simulink model "Q2_Vehicle_Steering_System"  (R2020a)
settings: Solver=VariableStepAuto  StartTime=0.0  StopTime=100  MaxStep=0.01  RelTol=1e-3
values from neighbouring files (symbols this model uses):
  A = [[0,1];[0,0]]    [Variables.m]
  B = [0.4; 1]    [Variables.m]
  C = eye(2)    [Variables.m]
  D = [0;0]    [Variables.m]
  K = [0.2500, 1.3]    [Variables.m]
  Kr = 0.25    [Variables.m]
  L = [2,1]    [Variables.m]
settings Model: Creator=Ajita Shree  LastModifiedBy=Ajita Shree

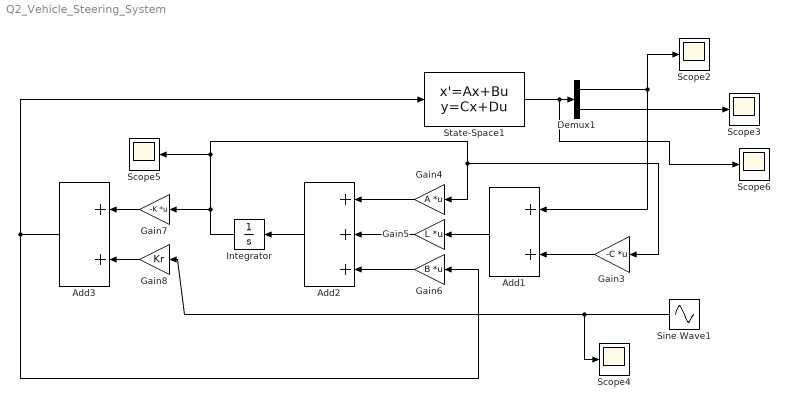
== system Q2_Vehicle_Steering_System ==
  Add1 : Sum
  Add2 : Sum  Inputs=+++
  Add3 : Sum
  Demux1 : Demux  Outputs=2
  Gain3 : Gain  Gain=-C  Multiplication=Matrix(K*u)
  Gain4 : Gain  Gain=A  Multiplication=Matrix(K*u)
  Gain5 : Gain  Gain=L  Multiplication=Matrix(K*u)
  Gain6 : Gain  Gain=B  Multiplication=Matrix(K*u)
  Gain7 : Gain  Gain=-K  Multiplication=Matrix(K*u)
  Gain8 : Gain  Gain=Kr
  Integrator : Integrator
  Scope{2..6} (5 alike) : Scope
  Sine Wave1 : Sin  Frequency=0.5  SampleTime=0
  State-Space1 : StateSpace  A=A  B=B  C=C  D=D  InitialCondition=0
  wires:
  State-Space1/1 -> Scope6/1, Demux1/1
  Demux1/1 -> Add1/1, Scope2/1
  Demux1/2 -> Scope3/1
  Gain4/1 -> Add2/1
  Gain5/1 -> Add2/2
  Gain6/1 -> Add2/3
  Add2/1 -> Integrator/1
  Integrator/1 -> Gain7/1, Gain4/1, Gain3/1, Scope5/1
  Gain3/1 -> Add1/2
  Add1/1 -> Gain5/1
  Add3/1 -> State-Space1/1, Gain6/1
  Gain7/1 -> Add3/1
  Gain8/1 -> Add3/2
  Sine Wave1/1 -> Scope4/1, Gain8/1
